simulink subsystem "rss_ComSpdFlt"  (R2023a)
settings: Solver=VariableStepAuto  StartTime=0.0  StopTime=10.0  RelTol=1e-3
undefined symbols (not defined in the file): bit, Cdbl_nElecAgSpdMaxVal
libraries: lib_configurable_parameter x1, lib_iir_filter x1
settings Model: Creator=xiaoqiang.yuan  LastModifiedBy=xiaoqiang.yuan

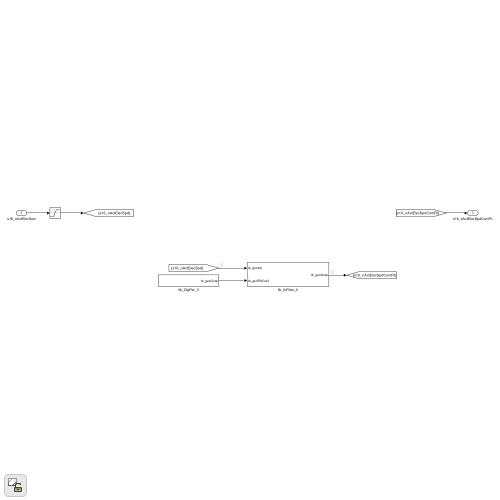
[thumbnail: Simulink's stored preview of the top-level diagram]
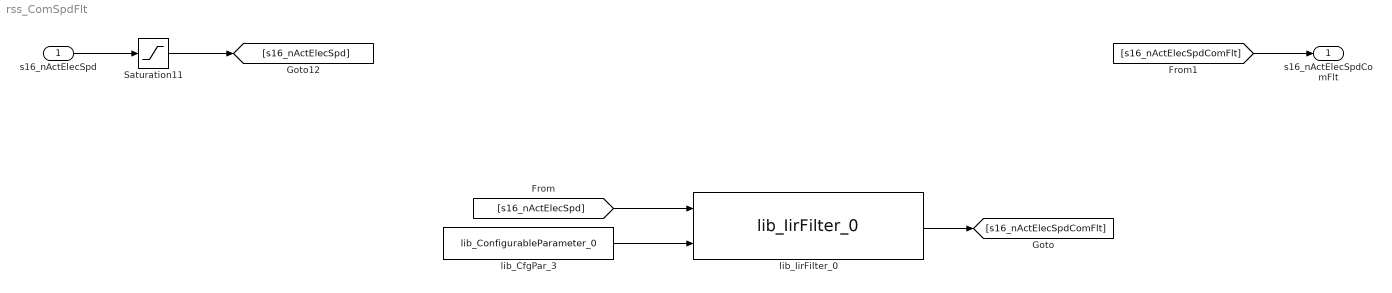
== system rss_ComSpdFlt ==
  s16_nActElecSpd : Inport  OutDataTypeStr=dt_Standardize_s16p15b0
  Saturation11 : Saturate  UpperLimit=Cdbl_nElecAgSpdMaxVal  LowerLimit=-Cdbl_nElecAgSpdMaxVal
  lib_CfgPar_3 : lib_configurable_parameter/lib_ConfigurableParameter_0  lb_parCnfgPar=Gu16_facComSpdFltCoeff_C  lb_parDataType=Inherit: Inherit from 'Constant value'  lb_parUpLim=Cdbl_facSpdFltCoeffMaxVal  lb_parLowLim=Cdbl_facSpdFltCoeffMinVal
  lib_IirFilter_0 : lib_iir_filter/lib_IirFilter_0  lb_parMaxInpVal=Cdbl_nElecAgSpdMaxVal  lb_parFltrCoefMaxVal=Cdbl_facSpdFltCoeffMaxVal  lb_parBitNumMode=16-bit  lb_parOutpDataType=dt_Standardize_s16p15b0  lb_parFiltTypeMode=Low-pass
  s16_nActElecSpdComFlt : Outport  OutDataTypeStr=dt_Standardize_s16p15b0
  wires:
  lib_CfgPar_3/1 -> lib_IirFilter_0/2
  Saturation11/1 -> [s16_nActElecSpd]
  s16_nActElecSpd/1 -> Saturation11/1
  [s16_nActElecSpd] -> lib_IirFilter_0/1
  [s16_nActElecSpdComFlt] -> s16_nActElecSpdComFlt/1
  lib_IirFilter_0/1 -> [s16_nActElecSpdComFlt]
